simulink library "Thermal_Capacity"  (Simulink 8.2)
settings: Solver=ode45  StartTime=0.0  StopTime=10.0  RelTol=1e-3
settings Model: Creator=drhf  LastModifiedBy=drhf

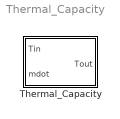
== system Thermal_Capacity ==
  Thermal_Capacity : Subsystem  mask(Thermal Capacity){UA=1, mcp=4182*10, Tamb=20, cp_approx=4000}
      mask prompts: UA "Loss coefficient in W/K"; mcp "Thermal capacity in J/K"; Tamb "Ambient temperature in °C"; cp_approx "heat capacity of fluid in J/kg/K (approximate value)"
      mask help: Basic one node model of a thermal mass using the differential equation:
      mask Help: web(fullfile(path_carnot('help'),'Thermal_Capacity.html'),'-helpbrowser')

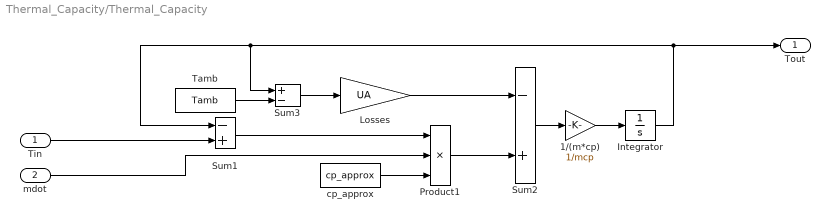
== system Thermal_Capacity/Thermal_Capacity ==
  Tin : Inport
  mdot : Inport  Port=2
  1/(m*cp) : Gain  Gain=1/mcp  SaturateOnIntegerOverflow=on  OutDataTypeStr=Inherit: Same as input  ParamDataTypeStr=Inherit: Same as input
  Integrator : Integrator  InitialCondition=Tamb
  Losses : Gain  Gain=UA  SaturateOnIntegerOverflow=on  OutDataTypeStr=Inherit: Same as input  ParamDataTypeStr=Inherit: Same as input
  Product1 : Product  Inputs=3  SaturateOnIntegerOverflow=on  InputSameDT=on  OutDataTypeStr=Inherit: Same as first input
  Sum1 : Sum  Inputs=-+  SaturateOnIntegerOverflow=on  InputSameDT=on  OutDataTypeStr=Inherit: Same as first input
  Sum2 : Sum  Inputs=-+  SaturateOnIntegerOverflow=on  InputSameDT=on  OutDataTypeStr=Inherit: Same as first input
  Sum3 : Sum  Inputs=+-  SaturateOnIntegerOverflow=on  InputSameDT=on  OutDataTypeStr=Inherit: Same as first input
  Tamb : Constant  Value=Tamb
  cp_approx : Constant  Value=cp_approx
  Tout : Outport
  wires:
  Sum1/1 -> Product1/1
  1/(m*cp)/1 -> Integrator/1
  cp_approx/1 -> Product1/3
  Sum3/1 -> Losses/1
  Losses/1 -> Sum2/1
  Tamb/1 -> Sum3/2
  Sum2/1 -> 1/(m*cp)/1
  Product1/1 -> Sum2/2
  Integrator/1 -> Tout/1, Sum3/1, Sum1/1
  Tin/1 -> Sum1/2
  mdot/1 -> Product1/2
